simulink model "LV_grid"  (R2019b)
settings: Solver=VariableStepAuto  StartTime=0  StopTime=5.005  FixedStep=5e-4  RelTol=1e-3
model workspace (MAT data in the model file):
  P2_1 = 3450
libraries: powerlib x373, powerlib_meascontrol x37
(part 3 of 5)

== system LV_grid/L20 ==
  note: 2.5m
  note: 2.5m
  note: 2.5m
  Ground : powerlib/Elements/Ground  LConnTagsString=a
      settings: SourceProductName=Simscape Electrical
  Ground1 : powerlib/Elements/Ground  LConnTagsString=a
      settings: SourceProductName=Simscape Electrical
  L1 : Subsystem
  L2 : Subsystem
  L3 : Subsystem
  A : PMIOPort  Side=Left
  B : PMIOPort  Port=2  Side=Left
  C : PMIOPort  Port=3  Side=Left
  N : PMIOPort  Port=4  Side=Left
  a : PMIOPort  Port=5  Side=Right
  b : PMIOPort  Port=6  Side=Right
  c : PMIOPort  Port=7  Side=Right
  n : PMIOPort  Port=8  Side=Right
  connections:
  L1/LConn2 -- B/RConn1
  L1/LConn4 -- N/RConn1
  L1/LConn1 -- A/RConn1
  L1/RConn4 -- L2/LConn4 -- Ground/LConn1
  L1/LConn3 -- C/RConn1
  L3/RConn4 -- n/RConn1
  L2/RConn4 -- L3/LConn4 -- Ground1/LConn1
  L3/RConn1 -- a/RConn1
  L3/RConn2 -- b/RConn1
  L3/RConn3 -- c/RConn1
  L3/LConn1 -- L2/RConn1
  L3/LConn2 -- L2/RConn2
  L3/LConn3 -- L2/RConn3
  L2/LConn1 -- L1/RConn1
  L2/LConn2 -- L1/RConn2
  L2/LConn3 -- L1/RConn3

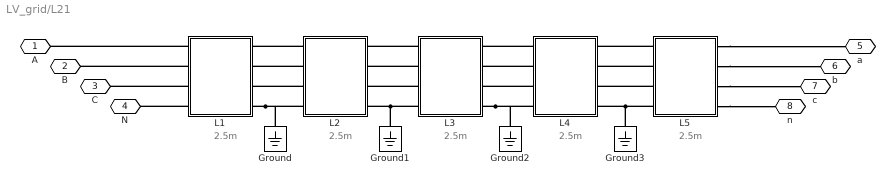
== system LV_grid/L21 ==
  note: 2.5m
  note: 2.5m
  note: 2.5m
  note: 2.5m
  note: 2.5m
  Ground{,1..3} (4 alike) : powerlib/Elements/Ground  LConnTagsString=a
      settings: SourceProductName=Simscape Electrical
  L1 : Subsystem
  L2 : Subsystem
  L3 : Subsystem
  L4 : Subsystem
  L5 : Subsystem
  A : PMIOPort  Side=Left
  B : PMIOPort  Port=2  Side=Left
  C : PMIOPort  Port=3  Side=Left
  N : PMIOPort  Port=4  Side=Left
  a : PMIOPort  Port=5  Side=Right
  b : PMIOPort  Port=6  Side=Right
  c : PMIOPort  Port=7  Side=Right
  n : PMIOPort  Port=8  Side=Right
  connections:
  L1/LConn1 -- A/RConn1
  L1/LConn4 -- N/RConn1
  L1/LConn2 -- B/RConn1
  L1/LConn3 -- C/RConn1
  L5/LConn4 -- L4/RConn4 -- Ground3/LConn1
  L3/RConn4 -- L4/LConn4 -- Ground2/LConn1
  L5/RConn4 -- n/RConn1
  L3/LConn4 -- L2/RConn4 -- Ground1/LConn1
  L1/RConn4 -- L2/LConn4 -- Ground/LConn1
  L5/RConn1 -- a/RConn1
  L5/RConn2 -- b/RConn1
  L5/RConn3 -- c/RConn1
  L2/LConn1 -- L1/RConn1
  L2/LConn2 -- L1/RConn2
  L2/LConn3 -- L1/RConn3
  L4/LConn1 -- L3/RConn1
  L4/LConn2 -- L3/RConn2
  L4/LConn3 -- L3/RConn3
  L5/LConn1 -- L4/RConn1
  L5/LConn2 -- L4/RConn2
  L5/LConn3 -- L4/RConn3
  L3/LConn1 -- L2/RConn1
  L3/LConn2 -- L2/RConn2
  L3/LConn3 -- L2/RConn3

== system LV_grid/L22 ==
  note: 2.5m
  note: 2.5m
  Ground : powerlib/Elements/Ground  LConnTagsString=a
      settings: SourceProductName=Simscape Electrical
  L1 : Subsystem
  L2 : Subsystem
  A : PMIOPort  Side=Left
  B : PMIOPort  Port=2  Side=Left
  C : PMIOPort  Port=3  Side=Left
  N : PMIOPort  Port=4  Side=Left
  a : PMIOPort  Port=5  Side=Right
  b : PMIOPort  Port=6  Side=Right
  c : PMIOPort  Port=7  Side=Right
  n : PMIOPort  Port=8  Side=Right
  connections:
  L2/RConn4 -- n/RConn1
  L1/RConn4 -- L2/LConn4 -- Ground/LConn1
  L1/LConn4 -- N/RConn1
  L1/LConn3 -- C/RConn1
  L1/LConn2 -- B/RConn1
  L1/LConn1 -- A/RConn1
  L2/LConn1 -- L1/RConn1
  L2/LConn2 -- L1/RConn2
  L2/LConn3 -- L1/RConn3
  L2/RConn1 -- a/RConn1
  L2/RConn2 -- b/RConn1
  L2/RConn3 -- c/RConn1

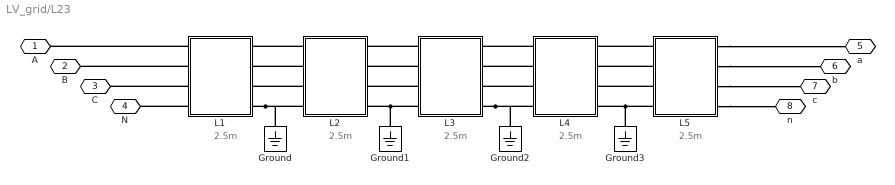
== system LV_grid/L23 ==
  note: 2.5m
  note: 2.5m
  note: 2.5m
  note: 2.5m
  note: 2.5m
  Ground{,1..3} (4 alike) : powerlib/Elements/Ground  LConnTagsString=a
      settings: SourceProductName=Simscape Electrical
  L1 : Subsystem
  L2 : Subsystem
  L3 : Subsystem
  L4 : Subsystem
  L5 : Subsystem
  A : PMIOPort  Side=Left
  B : PMIOPort  Port=2  Side=Left
  C : PMIOPort  Port=3  Side=Left
  N : PMIOPort  Port=4  Side=Left
  a : PMIOPort  Port=5  Side=Right
  b : PMIOPort  Port=6  Side=Right
  c : PMIOPort  Port=7  Side=Right
  n : PMIOPort  Port=8  Side=Right
  connections:
  L1/LConn1 -- A/RConn1
  L1/LConn4 -- N/RConn1
  L1/LConn2 -- B/RConn1
  L1/LConn3 -- C/RConn1
  L5/LConn4 -- L4/RConn4 -- Ground3/LConn1
  L3/RConn4 -- L4/LConn4 -- Ground2/LConn1
  L5/RConn4 -- n/RConn1
  L3/LConn4 -- L2/RConn4 -- Ground1/LConn1
  L1/RConn4 -- L2/LConn4 -- Ground/LConn1
  L4/LConn1 -- L3/RConn1
  L4/LConn2 -- L3/RConn2
  L4/LConn3 -- L3/RConn3
  L2/LConn1 -- L1/RConn1
  L2/LConn2 -- L1/RConn2
  L2/LConn3 -- L1/RConn3
  L5/RConn1 -- a/RConn1
  L5/RConn2 -- b/RConn1
  L5/RConn3 -- c/RConn1
  L5/LConn1 -- L4/RConn1
  L5/LConn2 -- L4/RConn2
  L5/LConn3 -- L4/RConn3
  L3/LConn1 -- L2/RConn1
  L3/LConn2 -- L2/RConn2
  L3/LConn3 -- L2/RConn3

== system LV_grid/L24 ==
  note: 2.5m
  note: 2.5m
  note: 2.5m
  note: 2.5m
  Ground : powerlib/Elements/Ground  LConnTagsString=a
      settings: SourceProductName=Simscape Electrical
  Ground1 : powerlib/Elements/Ground  LConnTagsString=a
      settings: SourceProductName=Simscape Electrical
  Ground2 : powerlib/Elements/Ground  LConnTagsString=a
      settings: SourceProductName=Simscape Electrical
  L1 : Subsystem
  L2 : Subsystem
  L3 : Subsystem
  L4 : Subsystem
  A : PMIOPort  Side=Left
  B : PMIOPort  Port=2  Side=Left
  C : PMIOPort  Port=3  Side=Left
  N : PMIOPort  Port=4  Side=Left
  a : PMIOPort  Port=5  Side=Right
  b : PMIOPort  Port=6  Side=Right
  c : PMIOPort  Port=7  Side=Right
  n : PMIOPort  Port=8  Side=Right
  connections:
  L1/LConn3 -- C/RConn1
  L2/RConn4 -- L3/LConn4 -- Ground1/LConn1
  L1/LConn4 -- N/RConn1
  L1/LConn2 -- B/RConn1
  L1/LConn1 -- A/RConn1
  L1/RConn4 -- L2/LConn4 -- Ground/LConn1
  L3/RConn4 -- L4/LConn4 -- Ground2/LConn1
  L4/RConn4 -- n/RConn1
  L4/RConn1 -- a/RConn1
  L4/RConn2 -- b/RConn1
  L4/RConn3 -- c/RConn1
  L3/LConn1 -- L2/RConn1
  L3/LConn2 -- L2/RConn2
  L3/LConn3 -- L2/RConn3
  L2/LConn1 -- L1/RConn1
  L2/LConn2 -- L1/RConn2
  L2/LConn3 -- L1/RConn3
  L4/LConn1 -- L3/RConn1
  L4/LConn2 -- L3/RConn2
  L4/LConn3 -- L3/RConn3

== system LV_grid/L25 ==
  note: 2.5m
  note: 2.5m
  note: 2.5m
  note: 2.5m
  Ground : powerlib/Elements/Ground  LConnTagsString=a
      settings: SourceProductName=Simscape Electrical
  Ground1 : powerlib/Elements/Ground  LConnTagsString=a
      settings: SourceProductName=Simscape Electrical
  Ground2 : powerlib/Elements/Ground  LConnTagsString=a
      settings: SourceProductName=Simscape Electrical
  L1 : Subsystem
  L2 : Subsystem
  L3 : Subsystem
  L4 : Subsystem
  A : PMIOPort  Side=Left
  B : PMIOPort  Port=2  Side=Left
  C : PMIOPort  Port=3  Side=Left
  N : PMIOPort  Port=4  Side=Left
  a : PMIOPort  Port=5  Side=Right
  b : PMIOPort  Port=6  Side=Right
  c : PMIOPort  Port=7  Side=Right
  n : PMIOPort  Port=8  Side=Right
  connections:
  L1/LConn3 -- C/RConn1
  L3/LConn4 -- Ground1/LConn1 -- L2/RConn4
  L1/LConn4 -- N/RConn1
  L1/LConn2 -- B/RConn1
  L1/LConn1 -- A/RConn1
  L2/LConn4 -- Ground/LConn1 -- L1/RConn4
  L4/LConn4 -- Ground2/LConn1 -- L3/RConn4
  L4/RConn4 -- n/RConn1
  L3/LConn1 -- L2/RConn1
  L3/LConn2 -- L2/RConn2
  L3/LConn3 -- L2/RConn3
  L4/LConn1 -- L3/RConn1
  L4/LConn2 -- L3/RConn2
  L4/LConn3 -- L3/RConn3
  L4/RConn1 -- a/RConn1
  L4/RConn2 -- b/RConn1
  L4/RConn3 -- c/RConn1
  L2/LConn1 -- L1/RConn1
  L2/LConn2 -- L1/RConn2
  L2/LConn3 -- L1/RConn3

== system LV_grid/L26 ==
  note: 2.5m
  note: 2.5m
  Ground : powerlib/Elements/Ground  LConnTagsString=a
      settings: SourceProductName=Simscape Electrical
  L1 : Subsystem
  L2 : Subsystem
  A : PMIOPort  Side=Left
  B : PMIOPort  Port=2  Side=Left
  C : PMIOPort  Port=3  Side=Left
  N : PMIOPort  Port=4  Side=Left
  a : PMIOPort  Port=5  Side=Right
  b : PMIOPort  Port=6  Side=Right
  c : PMIOPort  Port=7  Side=Right
  n : PMIOPort  Port=8  Side=Right
  connections:
  L2/RConn4 -- n/RConn1
  L1/RConn4 -- L2/LConn4 -- Ground/LConn1
  L1/LConn4 -- N/RConn1
  L1/LConn3 -- C/RConn1
  L1/LConn2 -- B/RConn1
  L1/LConn1 -- A/RConn1
  L2/RConn1 -- a/RConn1
  L2/RConn2 -- b/RConn1
  L2/RConn3 -- c/RConn1
  L2/LConn1 -- L1/RConn1
  L2/LConn2 -- L1/RConn2
  L2/LConn3 -- L1/RConn3

== system LV_grid/L27 ==
  note: 2.5m
  note: 2.5m
  Ground : powerlib/Elements/Ground  LConnTagsString=a
      settings: SourceProductName=Simscape Electrical
  L1 : Subsystem
  L2 : Subsystem
  A : PMIOPort  Side=Left
  B : PMIOPort  Port=2  Side=Left
  C : PMIOPort  Port=3  Side=Left
  N : PMIOPort  Port=4  Side=Left
  a : PMIOPort  Port=5  Side=Right
  b : PMIOPort  Port=6  Side=Right
  c : PMIOPort  Port=7  Side=Right
  n : PMIOPort  Port=8  Side=Right
  connections:
  L2/RConn4 -- n/RConn1
  L1/RConn4 -- L2/LConn4 -- Ground/LConn1
  L1/LConn4 -- N/RConn1
  L1/LConn3 -- C/RConn1
  L1/LConn2 -- B/RConn1
  L1/LConn1 -- A/RConn1
  L2/RConn1 -- a/RConn1
  L2/RConn2 -- b/RConn1
  L2/RConn3 -- c/RConn1
  L2/LConn1 -- L1/RConn1
  L2/LConn2 -- L1/RConn2
  L2/LConn3 -- L1/RConn3

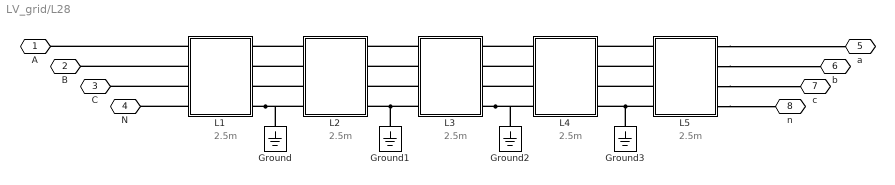
== system LV_grid/L28 ==
  note: 2.5m
  note: 2.5m
  note: 2.5m
  note: 2.5m
  note: 2.5m
  Ground{,1..3} (4 alike) : powerlib/Elements/Ground  LConnTagsString=a
      settings: SourceProductName=Simscape Electrical
  L1 : Subsystem
  L2 : Subsystem
  L3 : Subsystem
  L4 : Subsystem
  L5 : Subsystem
  A : PMIOPort  Side=Left
  B : PMIOPort  Port=2  Side=Left
  C : PMIOPort  Port=3  Side=Left
  N : PMIOPort  Port=4  Side=Left
  a : PMIOPort  Port=5  Side=Right
  b : PMIOPort  Port=6  Side=Right
  c : PMIOPort  Port=7  Side=Right
  n : PMIOPort  Port=8  Side=Right
  connections:
  L1/LConn1 -- A/RConn1
  L1/LConn4 -- N/RConn1
  L1/LConn2 -- B/RConn1
  L1/LConn3 -- C/RConn1
  L5/LConn4 -- L4/RConn4 -- Ground3/LConn1
  L3/RConn4 -- L4/LConn4 -- Ground2/LConn1
  L5/RConn4 -- n/RConn1
  L3/LConn4 -- L2/RConn4 -- Ground1/LConn1
  L1/RConn4 -- L2/LConn4 -- Ground/LConn1
  L3/LConn1 -- L2/RConn1
  L3/LConn2 -- L2/RConn2
  L3/LConn3 -- L2/RConn3
  L5/RConn1 -- a/RConn1
  L5/RConn2 -- b/RConn1
  L5/RConn3 -- c/RConn1
  L5/LConn1 -- L4/RConn1
  L5/LConn2 -- L4/RConn2
  L5/LConn3 -- L4/RConn3
  L4/LConn1 -- L3/RConn1
  L4/LConn2 -- L3/RConn2
  L4/LConn3 -- L3/RConn3
  L2/LConn1 -- L1/RConn1
  L2/LConn2 -- L1/RConn2
  L2/LConn3 -- L1/RConn3

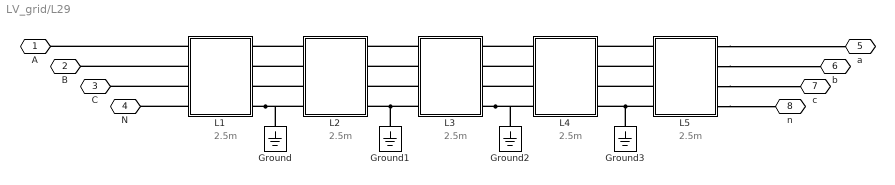
== system LV_grid/L29 ==
  note: 2.5m
  note: 2.5m
  note: 2.5m
  note: 2.5m
  note: 2.5m
  Ground{,1..3} (4 alike) : powerlib/Elements/Ground  LConnTagsString=a
      settings: SourceProductName=Simscape Electrical
  L1 : Subsystem
  L2 : Subsystem
  L3 : Subsystem
  L4 : Subsystem
  L5 : Subsystem
  A : PMIOPort  Side=Left
  B : PMIOPort  Port=2  Side=Left
  C : PMIOPort  Port=3  Side=Left
  N : PMIOPort  Port=4  Side=Left
  a : PMIOPort  Port=5  Side=Right
  b : PMIOPort  Port=6  Side=Right
  c : PMIOPort  Port=7  Side=Right
  n : PMIOPort  Port=8  Side=Right
  connections:
  L1/LConn1 -- A/RConn1
  L1/LConn4 -- N/RConn1
  L1/LConn2 -- B/RConn1
  L1/LConn3 -- C/RConn1
  L5/LConn4 -- L4/RConn4 -- Ground3/LConn1
  L3/RConn4 -- L4/LConn4 -- Ground2/LConn1
  L5/RConn4 -- n/RConn1
  L3/LConn4 -- L2/RConn4 -- Ground1/LConn1
  L1/RConn4 -- L2/LConn4 -- Ground/LConn1
  L4/LConn1 -- L3/RConn1
  L4/LConn2 -- L3/RConn2
  L4/LConn3 -- L3/RConn3
  L5/LConn1 -- L4/RConn1
  L5/LConn2 -- L4/RConn2
  L5/LConn3 -- L4/RConn3
  L2/LConn1 -- L1/RConn1
  L2/LConn2 -- L1/RConn2
  L2/LConn3 -- L1/RConn3
  L5/RConn1 -- a/RConn1
  L5/RConn2 -- b/RConn1
  L5/RConn3 -- c/RConn1
  L3/LConn1 -- L2/RConn1
  L3/LConn2 -- L2/RConn2
  L3/LConn3 -- L2/RConn3

== system LV_grid/L3 ==
  note: 2.5m
  L1 : Subsystem
  A : PMIOPort  Side=Left
  B : PMIOPort  Port=2  Side=Left
  C : PMIOPort  Port=3  Side=Left
  N : PMIOPort  Port=4  Side=Left
  a : PMIOPort  Port=5  Side=Right
  b : PMIOPort  Port=6  Side=Right
  c : PMIOPort  Port=7  Side=Right
  n : PMIOPort  Port=8  Side=Right
  connections:
  B/RConn1 -- L1/LConn2
  n/RConn1 -- L1/RConn4
  C/RConn1 -- L1/LConn3
  N/RConn1 -- L1/LConn4
  A/RConn1 -- L1/LConn1
  L1/RConn1 -- a/RConn1
  L1/RConn2 -- b/RConn1
  L1/RConn3 -- c/RConn1

== system LV_grid/L30 ==
  note: 2.5m
  note: 2.5m
  Ground : powerlib/Elements/Ground  LConnTagsString=a
      settings: SourceProductName=Simscape Electrical
  L1 : Subsystem
  L2 : Subsystem
  A : PMIOPort  Side=Left
  B : PMIOPort  Port=2  Side=Left
  C : PMIOPort  Port=3  Side=Left
  N : PMIOPort  Port=4  Side=Left
  a : PMIOPort  Port=5  Side=Right
  b : PMIOPort  Port=6  Side=Right
  c : PMIOPort  Port=7  Side=Right
  n : PMIOPort  Port=8  Side=Right
  connections:
  L2/RConn4 -- n/RConn1
  L1/RConn4 -- L2/LConn4 -- Ground/LConn1
  L1/LConn4 -- N/RConn1
  L1/LConn3 -- C/RConn1
  L1/LConn2 -- B/RConn1
  L1/LConn1 -- A/RConn1
  L2/LConn1 -- L1/RConn1
  L2/LConn2 -- L1/RConn2
  L2/LConn3 -- L1/RConn3
  L2/RConn1 -- a/RConn1
  L2/RConn2 -- b/RConn1
  L2/RConn3 -- c/RConn1

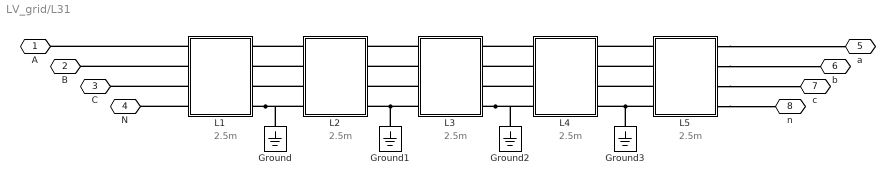
== system LV_grid/L31 ==
  note: 2.5m
  note: 2.5m
  note: 2.5m
  note: 2.5m
  note: 2.5m
  Ground{,1..3} (4 alike) : powerlib/Elements/Ground  LConnTagsString=a
      settings: SourceProductName=Simscape Electrical
  L1 : Subsystem
  L2 : Subsystem
  L3 : Subsystem
  L4 : Subsystem
  L5 : Subsystem
  A : PMIOPort  Side=Left
  B : PMIOPort  Port=2  Side=Left
  C : PMIOPort  Port=3  Side=Left
  N : PMIOPort  Port=4  Side=Left
  a : PMIOPort  Port=5  Side=Right
  b : PMIOPort  Port=6  Side=Right
  c : PMIOPort  Port=7  Side=Right
  n : PMIOPort  Port=8  Side=Right
  connections:
  L1/LConn1 -- A/RConn1
  L1/LConn4 -- N/RConn1
  L1/LConn2 -- B/RConn1
  L1/LConn3 -- C/RConn1
  L5/LConn4 -- L4/RConn4 -- Ground3/LConn1
  L3/RConn4 -- L4/LConn4 -- Ground2/LConn1
  L5/RConn4 -- n/RConn1
  L3/LConn4 -- L2/RConn4 -- Ground1/LConn1
  L1/RConn4 -- L2/LConn4 -- Ground/LConn1
  L5/RConn1 -- a/RConn1
  L5/RConn2 -- b/RConn1
  L5/RConn3 -- c/RConn1
  L3/LConn1 -- L2/RConn1
  L3/LConn2 -- L2/RConn2
  L3/LConn3 -- L2/RConn3
  L2/LConn1 -- L1/RConn1
  L2/LConn2 -- L1/RConn2
  L2/LConn3 -- L1/RConn3
  L5/LConn1 -- L4/RConn1
  L5/LConn2 -- L4/RConn2
  L5/LConn3 -- L4/RConn3
  L4/LConn1 -- L3/RConn1
  L4/LConn2 -- L3/RConn2
  L4/LConn3 -- L3/RConn3

== system LV_grid/L32 ==
  note: 2.5m
  note: 2.5m
  note: 2.5m
  note: 2.5m
  Ground : powerlib/Elements/Ground  LConnTagsString=a
      settings: SourceProductName=Simscape Electrical
  Ground1 : powerlib/Elements/Ground  LConnTagsString=a
      settings: SourceProductName=Simscape Electrical
  Ground2 : powerlib/Elements/Ground  LConnTagsString=a
      settings: SourceProductName=Simscape Electrical
  L1 : Subsystem
  L2 : Subsystem
  L3 : Subsystem
  L4 : Subsystem
  A : PMIOPort  Side=Left
  B : PMIOPort  Port=2  Side=Left
  C : PMIOPort  Port=3  Side=Left
  N : PMIOPort  Port=4  Side=Left
  a : PMIOPort  Port=5  Side=Right
  b : PMIOPort  Port=6  Side=Right
  c : PMIOPort  Port=7  Side=Right
  n : PMIOPort  Port=8  Side=Right
  connections:
  L1/LConn3 -- C/RConn1
  L2/RConn4 -- L3/LConn4 -- Ground1/LConn1
  L1/LConn4 -- N/RConn1
  L1/LConn2 -- B/RConn1
  L1/LConn1 -- A/RConn1
  L1/RConn4 -- L2/LConn4 -- Ground/LConn1
  L3/RConn4 -- L4/LConn4 -- Ground2/LConn1
  L4/RConn4 -- n/RConn1
  L4/RConn1 -- a/RConn1
  L4/RConn2 -- b/RConn1
  L4/RConn3 -- c/RConn1
  L2/LConn1 -- L1/RConn1
  L2/LConn2 -- L1/RConn2
  L2/LConn3 -- L1/RConn3
  L4/LConn1 -- L3/RConn1
  L4/LConn2 -- L3/RConn2
  L4/LConn3 -- L3/RConn3
  L3/LConn1 -- L2/RConn1
  L3/LConn2 -- L2/RConn2
  L3/LConn3 -- L2/RConn3

== system LV_grid/L4 ==
  note: 2.5m
  note: 2.5m
  Ground : powerlib/Elements/Ground  LConnTagsString=a
      settings: SourceProductName=Simscape Electrical
  L1 : Subsystem
  L2 : Subsystem
  A : PMIOPort  Side=Left
  B : PMIOPort  Port=2  Side=Left
  C : PMIOPort  Port=3  Side=Left
  N : PMIOPort  Port=4  Side=Left
  a : PMIOPort  Port=5  Side=Right
  b : PMIOPort  Port=6  Side=Right
  c : PMIOPort  Port=7  Side=Right
  n : PMIOPort  Port=8  Side=Right
  connections:
  L2/RConn4 -- n/RConn1
  L2/LConn4 -- Ground/LConn1 -- L1/RConn4
  L1/LConn4 -- N/RConn1
  L1/LConn3 -- C/RConn1
  L1/LConn2 -- B/RConn1
  L1/LConn1 -- A/RConn1
  L2/LConn1 -- L1/RConn1
  L2/LConn2 -- L1/RConn2
  L2/LConn3 -- L1/RConn3
  L2/RConn1 -- a/RConn1
  L2/RConn2 -- b/RConn1
  L2/RConn3 -- c/RConn1

== system LV_grid/L5 ==
  note: 2.5m
  note: 2.5m
  Ground : powerlib/Elements/Ground  LConnTagsString=a
      settings: SourceProductName=Simscape Electrical
  L1 : Subsystem
  L2 : Subsystem
  A : PMIOPort  Side=Left
  B : PMIOPort  Port=2  Side=Left
  C : PMIOPort  Port=3  Side=Left
  N : PMIOPort  Port=4  Side=Left
  a : PMIOPort  Port=5  Side=Right
  b : PMIOPort  Port=6  Side=Right
  c : PMIOPort  Port=7  Side=Right
  n : PMIOPort  Port=8  Side=Right
  connections:
  L2/RConn4 -- n/RConn1
  L1/RConn4 -- L2/LConn4 -- Ground/LConn1
  L1/LConn4 -- N/RConn1
  L1/LConn3 -- C/RConn1
  L1/LConn2 -- B/RConn1
  L1/LConn1 -- A/RConn1
  L2/LConn1 -- L1/RConn1
  L2/LConn2 -- L1/RConn2
  L2/LConn3 -- L1/RConn3
  L2/RConn1 -- a/RConn1
  L2/RConn2 -- b/RConn1
  L2/RConn3 -- c/RConn1

== system LV_grid/L6 ==
  note: 2.5m
  L1 : Subsystem
  A : PMIOPort  Side=Left
  B : PMIOPort  Port=2  Side=Left
  C : PMIOPort  Port=3  Side=Left
  N : PMIOPort  Port=4  Side=Left
  a : PMIOPort  Port=5  Side=Right
  b : PMIOPort  Port=6  Side=Right
  c : PMIOPort  Port=7  Side=Right
  n : PMIOPort  Port=8  Side=Right
  connections:
  B/RConn1 -- L1/LConn2
  n/RConn1 -- L1/RConn4
  C/RConn1 -- L1/LConn3
  N/RConn1 -- L1/LConn4
  A/RConn1 -- L1/LConn1
  L1/RConn1 -- a/RConn1
  L1/RConn2 -- b/RConn1
  L1/RConn3 -- c/RConn1

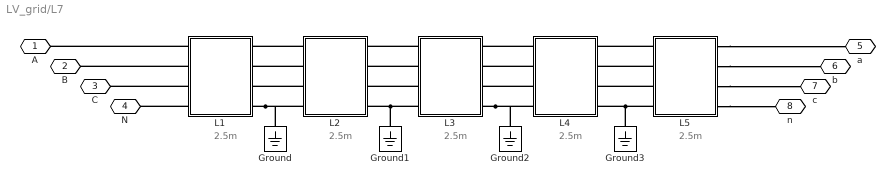
== system LV_grid/L7 ==
  note: 2.5m
  note: 2.5m
  note: 2.5m
  note: 2.5m
  note: 2.5m
  Ground{,1..3} (4 alike) : powerlib/Elements/Ground  LConnTagsString=a
      settings: SourceProductName=Simscape Electrical
  L1 : Subsystem
  L2 : Subsystem
  L3 : Subsystem
  L4 : Subsystem
  L5 : Subsystem
  A : PMIOPort  Side=Left
  B : PMIOPort  Port=2  Side=Left
  C : PMIOPort  Port=3  Side=Left
  N : PMIOPort  Port=4  Side=Left
  a : PMIOPort  Port=5  Side=Right
  b : PMIOPort  Port=6  Side=Right
  c : PMIOPort  Port=7  Side=Right
  n : PMIOPort  Port=8  Side=Right
  connections:
  L1/LConn1 -- A/RConn1
  L1/LConn4 -- N/RConn1
  L1/LConn2 -- B/RConn1
  L1/LConn3 -- C/RConn1
  L5/LConn4 -- L4/RConn4 -- Ground3/LConn1
  L3/RConn4 -- L4/LConn4 -- Ground2/LConn1
  L5/RConn4 -- n/RConn1
  L3/LConn4 -- L2/RConn4 -- Ground1/LConn1
  L1/RConn4 -- L2/LConn4 -- Ground/LConn1
  L3/LConn1 -- L2/RConn1
  L3/LConn2 -- L2/RConn2
  L3/LConn3 -- L2/RConn3
  L5/LConn1 -- L4/RConn1
  L5/LConn2 -- L4/RConn2
  L5/LConn3 -- L4/RConn3
  L5/RConn1 -- a/RConn1
  L5/RConn2 -- b/RConn1
  L5/RConn3 -- c/RConn1
  L4/LConn1 -- L3/RConn1
  L4/LConn2 -- L3/RConn2
  L4/LConn3 -- L3/RConn3
  L2/LConn1 -- L1/RConn1
  L2/LConn2 -- L1/RConn2
  L2/LConn3 -- L1/RConn3

== system LV_grid/L8 ==
  note: 2.5m
  note: 2.5m
  note: 2.5m
  Ground : powerlib/Elements/Ground  LConnTagsString=a
      settings: SourceProductName=Simscape Electrical
  Ground1 : powerlib/Elements/Ground  LConnTagsString=a
      settings: SourceProductName=Simscape Electrical
  L1 : Subsystem
  L2 : Subsystem
  L3 : Subsystem
  A : PMIOPort  Side=Left
  B : PMIOPort  Port=2  Side=Left
  C : PMIOPort  Port=3  Side=Left
  N : PMIOPort  Port=4  Side=Left
  a : PMIOPort  Port=5  Side=Right
  b : PMIOPort  Port=6  Side=Right
  c : PMIOPort  Port=7  Side=Right
  n : PMIOPort  Port=8  Side=Right
  connections:
  L1/LConn2 -- B/RConn1
  L1/LConn4 -- N/RConn1
  L1/LConn1 -- A/RConn1
  L2/LConn4 -- Ground/LConn1 -- L1/RConn4
  L1/LConn3 -- C/RConn1
  L3/RConn4 -- n/RConn1
  L3/LConn4 -- Ground1/LConn1 -- L2/RConn4
  L3/RConn1 -- a/RConn1
  L3/RConn2 -- b/RConn1
  L3/RConn3 -- c/RConn1
  L3/LConn1 -- L2/RConn1
  L3/LConn2 -- L2/RConn2
  L3/LConn3 -- L2/RConn3
  L2/LConn1 -- L1/RConn1
  L2/LConn2 -- L1/RConn2
  L2/LConn3 -- L1/RConn3

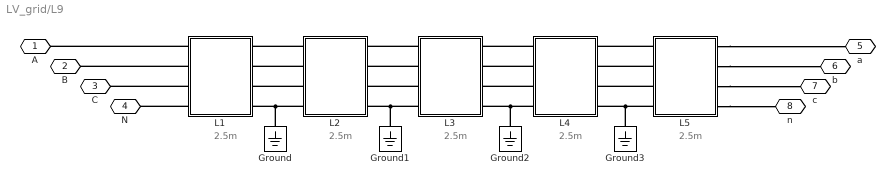
== system LV_grid/L9 ==
  note: 2.5m
  note: 2.5m
  note: 2.5m
  note: 2.5m
  note: 2.5m
  Ground{,1..3} (4 alike) : powerlib/Elements/Ground  LConnTagsString=a
      settings: SourceProductName=Simscape Electrical
  L1 : Subsystem
  L2 : Subsystem
  L3 : Subsystem
  L4 : Subsystem
  L5 : Subsystem
  A : PMIOPort  Side=Left
  B : PMIOPort  Port=2  Side=Left
  C : PMIOPort  Port=3  Side=Left
  N : PMIOPort  Port=4  Side=Left
  a : PMIOPort  Port=5  Side=Right
  b : PMIOPort  Port=6  Side=Right
  c : PMIOPort  Port=7  Side=Right
  n : PMIOPort  Port=8  Side=Right
  connections:
  L1/LConn1 -- A/RConn1
  L1/LConn4 -- N/RConn1
  L1/LConn2 -- B/RConn1
  L1/LConn3 -- C/RConn1
  L5/LConn4 -- Ground3/LConn1 -- L4/RConn4
  L4/LConn4 -- Ground2/LConn1 -- L3/RConn4
  L5/RConn4 -- n/RConn1
  L3/LConn4 -- Ground1/LConn1 -- L2/RConn4
  L2/LConn4 -- Ground/LConn1 -- L1/RConn4
  L5/LConn1 -- L4/RConn1
  L5/LConn2 -- L4/RConn2
  L5/LConn3 -- L4/RConn3
  L5/RConn1 -- a/RConn1
  L5/RConn2 -- b/RConn1
  L5/RConn3 -- c/RConn1
  L4/LConn1 -- L3/RConn1
  L4/LConn2 -- L3/RConn2
  L4/LConn3 -- L3/RConn3
  L2/LConn1 -- L1/RConn1
  L2/LConn2 -- L1/RConn2
  L2/LConn3 -- L1/RConn3
  L3/LConn1 -- L2/RConn1
  L3/LConn2 -- L2/RConn2
  L3/LConn3 -- L2/RConn3

== system LV_grid/L1/L1 ==
  Pi Section Line : powerlib/Elements/Pi Section Line  LConnTagsString=__new0  RConnTagsString=__new0  Frequency=50  Resistance=0.274  Inductance=0.073  Capacitance=12.74e-9  Length=0.0025  PiSections=1  Measurements=None
      settings: AttributesFormatString=\n  SourceProductName=Simscape Electrical  SourceProductBaseCode=PS
  Three-Phase PI Section Line : powerlib/Elements/Three-Phase PI Section Line  LConnTagsString=a|b|c  RConnTagsString=A|B|C  Frequency=50  Resistances=[ 0.274 0.959]  Inductances=[ 0.073 0.079]  Capacitances=[12.74e-9 7.751e-9]  Length=0.0025
      settings: SourceProductName=Simscape Electrical
  A : PMIOPort  Side=Left
  B : PMIOPort  Port=2  Side=Left
  C : PMIOPort  Port=3  Side=Left
  N : PMIOPort  Port=4  Side=Left
  a : PMIOPort  Port=5  Side=Right
  b : PMIOPort  Port=6  Side=Right
  c : PMIOPort  Port=7  Side=Right
  n : PMIOPort  Port=8  Side=Right
  connections:
  Pi Section Line/LConn1 -- N/RConn1
  Pi Section Line/RConn1 -- n/RConn1
  C/RConn1 -- Three-Phase PI Section Line/LConn3
  B/RConn1 -- Three-Phase PI Section Line/LConn2
  A/RConn1 -- Three-Phase PI Section Line/LConn1
  Three-Phase PI Section Line/RConn3 -- c/RConn1
  Three-Phase PI Section Line/RConn2 -- b/RConn1
  Three-Phase PI Section Line/RConn1 -- a/RConn1

== system LV_grid/L10/L1 ==
  Pi Section Line : powerlib/Elements/Pi Section Line  LConnTagsString=__new0  RConnTagsString=__new0  Frequency=50  Resistance=0.274  Inductance=0.073  Capacitance=12.74e-9  Length=0.0025  PiSections=1  Measurements=None
      settings: AttributesFormatString=\n  SourceProductName=Simscape Electrical  SourceProductBaseCode=PS
  Three-Phase PI Section Line : powerlib/Elements/Three-Phase PI Section Line  LConnTagsString=a|b|c  RConnTagsString=A|B|C  Frequency=50  Resistances=[ 0.274 0.959]  Inductances=[ 0.073 0.079]  Capacitances=[12.74e-9 7.751e-9]  Length=0.0025
      settings: SourceProductName=Simscape Electrical
  A : PMIOPort  Side=Left
  B : PMIOPort  Port=2  Side=Left
  C : PMIOPort  Port=3  Side=Left
  N : PMIOPort  Port=4  Side=Left
  a : PMIOPort  Port=5  Side=Right
  b : PMIOPort  Port=6  Side=Right
  c : PMIOPort  Port=7  Side=Right
  n : PMIOPort  Port=8  Side=Right
  connections:
  Pi Section Line/LConn1 -- N/RConn1
  Pi Section Line/RConn1 -- n/RConn1
  C/RConn1 -- Three-Phase PI Section Line/LConn3
  B/RConn1 -- Three-Phase PI Section Line/LConn2
  A/RConn1 -- Three-Phase PI Section Line/LConn1
  Three-Phase PI Section Line/RConn3 -- c/RConn1
  Three-Phase PI Section Line/RConn2 -- b/RConn1
  Three-Phase PI Section Line/RConn1 -- a/RConn1

== system LV_grid/L10/L2 ==
  Pi Section Line : powerlib/Elements/Pi Section Line  LConnTagsString=__new0  RConnTagsString=__new0  Frequency=50  Resistance=0.274  Inductance=0.073  Capacitance=12.74e-9  Length=0.0025  PiSections=1  Measurements=None
      settings: AttributesFormatString=\n  SourceProductName=Simscape Electrical  SourceProductBaseCode=PS
  Three-Phase PI Section Line : powerlib/Elements/Three-Phase PI Section Line  LConnTagsString=a|b|c  RConnTagsString=A|B|C  Frequency=50  Resistances=[ 0.274 0.959]  Inductances=[ 0.073 0.079]  Capacitances=[12.74e-9 7.751e-9]  Length=0.0025
      settings: SourceProductName=Simscape Electrical
  A : PMIOPort  Side=Left
  B : PMIOPort  Port=2  Side=Left
  C : PMIOPort  Port=3  Side=Left
  N : PMIOPort  Port=4  Side=Left
  a : PMIOPort  Port=5  Side=Right
  b : PMIOPort  Port=6  Side=Right
  c : PMIOPort  Port=7  Side=Right
  n : PMIOPort  Port=8  Side=Right
  connections:
  Pi Section Line/LConn1 -- N/RConn1
  Pi Section Line/RConn1 -- n/RConn1
  C/RConn1 -- Three-Phase PI Section Line/LConn3
  B/RConn1 -- Three-Phase PI Section Line/LConn2
  A/RConn1 -- Three-Phase PI Section Line/LConn1
  Three-Phase PI Section Line/RConn3 -- c/RConn1
  Three-Phase PI Section Line/RConn2 -- b/RConn1
  Three-Phase PI Section Line/RConn1 -- a/RConn1

== system LV_grid/L11/L1 ==
  Pi Section Line : powerlib/Elements/Pi Section Line  LConnTagsString=__new0  RConnTagsString=__new0  Frequency=50  Resistance=0.274  Inductance=0.073  Capacitance=12.74e-9  Length=0.0025  PiSections=1  Measurements=None
      settings: AttributesFormatString=\n  SourceProductName=Simscape Electrical  SourceProductBaseCode=PS
  Three-Phase PI Section Line : powerlib/Elements/Three-Phase PI Section Line  LConnTagsString=a|b|c  RConnTagsString=A|B|C  Frequency=50  Resistances=[ 0.274 0.959]  Inductances=[ 0.073 0.079]  Capacitances=[12.74e-9 7.751e-9]  Length=0.0025
      settings: SourceProductName=Simscape Electrical
  A : PMIOPort  Side=Left
  B : PMIOPort  Port=2  Side=Left
  C : PMIOPort  Port=3  Side=Left
  N : PMIOPort  Port=4  Side=Left
  a : PMIOPort  Port=5  Side=Right
  b : PMIOPort  Port=6  Side=Right
  c : PMIOPort  Port=7  Side=Right
  n : PMIOPort  Port=8  Side=Right
  connections:
  Pi Section Line/LConn1 -- N/RConn1
  Pi Section Line/RConn1 -- n/RConn1
  C/RConn1 -- Three-Phase PI Section Line/LConn3
  B/RConn1 -- Three-Phase PI Section Line/LConn2
  A/RConn1 -- Three-Phase PI Section Line/LConn1
  Three-Phase PI Section Line/RConn3 -- c/RConn1
  Three-Phase PI Section Line/RConn2 -- b/RConn1
  Three-Phase PI Section Line/RConn1 -- a/RConn1

== system LV_grid/L11/L2 ==
  Pi Section Line : powerlib/Elements/Pi Section Line  LConnTagsString=__new0  RConnTagsString=__new0  Frequency=50  Resistance=0.274  Inductance=0.073  Capacitance=12.74e-9  Length=0.0025  PiSections=1  Measurements=None
      settings: AttributesFormatString=\n  SourceProductName=Simscape Electrical  SourceProductBaseCode=PS
  Three-Phase PI Section Line : powerlib/Elements/Three-Phase PI Section Line  LConnTagsString=a|b|c  RConnTagsString=A|B|C  Frequency=50  Resistances=[ 0.274 0.959]  Inductances=[ 0.073 0.079]  Capacitances=[12.74e-9 7.751e-9]  Length=0.0025
      settings: SourceProductName=Simscape Electrical
  A : PMIOPort  Side=Left
  B : PMIOPort  Port=2  Side=Left
  C : PMIOPort  Port=3  Side=Left
  N : PMIOPort  Port=4  Side=Left
  a : PMIOPort  Port=5  Side=Right
  b : PMIOPort  Port=6  Side=Right
  c : PMIOPort  Port=7  Side=Right
  n : PMIOPort  Port=8  Side=Right
  connections:
  Pi Section Line/LConn1 -- N/RConn1
  Pi Section Line/RConn1 -- n/RConn1
  C/RConn1 -- Three-Phase PI Section Line/LConn3
  B/RConn1 -- Three-Phase PI Section Line/LConn2
  A/RConn1 -- Three-Phase PI Section Line/LConn1
  Three-Phase PI Section Line/RConn3 -- c/RConn1
  Three-Phase PI Section Line/RConn2 -- b/RConn1
  Three-Phase PI Section Line/RConn1 -- a/RConn1

== system LV_grid/L12/L1 ==
  Pi Section Line : powerlib/Elements/Pi Section Line  LConnTagsString=__new0  RConnTagsString=__new0  Frequency=50  Resistance=0.274  Inductance=0.073  Capacitance=12.74e-9  Length=0.0025  PiSections=1  Measurements=None
      settings: AttributesFormatString=\n  SourceProductName=Simscape Electrical  SourceProductBaseCode=PS
  Three-Phase PI Section Line : powerlib/Elements/Three-Phase PI Section Line  LConnTagsString=a|b|c  RConnTagsString=A|B|C  Frequency=50  Resistances=[ 0.274 0.959]  Inductances=[ 0.073 0.079]  Capacitances=[12.74e-9 7.751e-9]  Length=0.0025
      settings: SourceProductName=Simscape Electrical
  A : PMIOPort  Side=Left
  B : PMIOPort  Port=2  Side=Left
  C : PMIOPort  Port=3  Side=Left
  N : PMIOPort  Port=4  Side=Left
  a : PMIOPort  Port=5  Side=Right
  b : PMIOPort  Port=6  Side=Right
  c : PMIOPort  Port=7  Side=Right
  n : PMIOPort  Port=8  Side=Right
  connections:
  Pi Section Line/LConn1 -- N/RConn1
  Pi Section Line/RConn1 -- n/RConn1
  C/RConn1 -- Three-Phase PI Section Line/LConn3
  B/RConn1 -- Three-Phase PI Section Line/LConn2
  A/RConn1 -- Three-Phase PI Section Line/LConn1
  Three-Phase PI Section Line/RConn3 -- c/RConn1
  Three-Phase PI Section Line/RConn2 -- b/RConn1
  Three-Phase PI Section Line/RConn1 -- a/RConn1

== system LV_grid/L12/L2 ==
  Pi Section Line : powerlib/Elements/Pi Section Line  LConnTagsString=__new0  RConnTagsString=__new0  Frequency=50  Resistance=0.274  Inductance=0.073  Capacitance=12.74e-9  Length=0.0025  PiSections=1  Measurements=None
      settings: AttributesFormatString=\n  SourceProductName=Simscape Electrical  SourceProductBaseCode=PS
  Three-Phase PI Section Line : powerlib/Elements/Three-Phase PI Section Line  LConnTagsString=a|b|c  RConnTagsString=A|B|C  Frequency=50  Resistances=[ 0.274 0.959]  Inductances=[ 0.073 0.079]  Capacitances=[12.74e-9 7.751e-9]  Length=0.0025
      settings: SourceProductName=Simscape Electrical
  A : PMIOPort  Side=Left
  B : PMIOPort  Port=2  Side=Left
  C : PMIOPort  Port=3  Side=Left
  N : PMIOPort  Port=4  Side=Left
  a : PMIOPort  Port=5  Side=Right
  b : PMIOPort  Port=6  Side=Right
  c : PMIOPort  Port=7  Side=Right
  n : PMIOPort  Port=8  Side=Right
  connections:
  Pi Section Line/LConn1 -- N/RConn1
  Pi Section Line/RConn1 -- n/RConn1
  C/RConn1 -- Three-Phase PI Section Line/LConn3
  B/RConn1 -- Three-Phase PI Section Line/LConn2
  A/RConn1 -- Three-Phase PI Section Line/LConn1
  Three-Phase PI Section Line/RConn3 -- c/RConn1
  Three-Phase PI Section Line/RConn2 -- b/RConn1
  Three-Phase PI Section Line/RConn1 -- a/RConn1

== system LV_grid/L12/L3 ==
  Pi Section Line : powerlib/Elements/Pi Section Line  LConnTagsString=__new0  RConnTagsString=__new0  Frequency=50  Resistance=0.274  Inductance=0.073  Capacitance=12.74e-9  Length=0.0025  PiSections=1  Measurements=None
      settings: AttributesFormatString=\n  SourceProductName=Simscape Electrical  SourceProductBaseCode=PS
  Three-Phase PI Section Line : powerlib/Elements/Three-Phase PI Section Line  LConnTagsString=a|b|c  RConnTagsString=A|B|C  Frequency=50  Resistances=[ 0.274 0.959]  Inductances=[ 0.073 0.079]  Capacitances=[12.74e-9 7.751e-9]  Length=0.0025
      settings: SourceProductName=Simscape Electrical
  A : PMIOPort  Side=Left
  B : PMIOPort  Port=2  Side=Left
  C : PMIOPort  Port=3  Side=Left
  N : PMIOPort  Port=4  Side=Left
  a : PMIOPort  Port=5  Side=Right
  b : PMIOPort  Port=6  Side=Right
  c : PMIOPort  Port=7  Side=Right
  n : PMIOPort  Port=8  Side=Right
  connections:
  Pi Section Line/LConn1 -- N/RConn1
  Pi Section Line/RConn1 -- n/RConn1
  C/RConn1 -- Three-Phase PI Section Line/LConn3
  B/RConn1 -- Three-Phase PI Section Line/LConn2
  A/RConn1 -- Three-Phase PI Section Line/LConn1
  Three-Phase PI Section Line/RConn3 -- c/RConn1
  Three-Phase PI Section Line/RConn2 -- b/RConn1
  Three-Phase PI Section Line/RConn1 -- a/RConn1

== system LV_grid/L12/L4 ==
  Pi Section Line : powerlib/Elements/Pi Section Line  LConnTagsString=__new0  RConnTagsString=__new0  Frequency=50  Resistance=0.274  Inductance=0.073  Capacitance=12.74e-9  Length=0.0025  PiSections=1  Measurements=None
      settings: AttributesFormatString=\n  SourceProductName=Simscape Electrical  SourceProductBaseCode=PS
  Three-Phase PI Section Line : powerlib/Elements/Three-Phase PI Section Line  LConnTagsString=a|b|c  RConnTagsString=A|B|C  Frequency=50  Resistances=[ 0.274 0.959]  Inductances=[ 0.073 0.079]  Capacitances=[12.74e-9 7.751e-9]  Length=0.0025
      settings: SourceProductName=Simscape Electrical
  A : PMIOPort  Side=Left
  B : PMIOPort  Port=2  Side=Left
  C : PMIOPort  Port=3  Side=Left
  N : PMIOPort  Port=4  Side=Left
  a : PMIOPort  Port=5  Side=Right
  b : PMIOPort  Port=6  Side=Right
  c : PMIOPort  Port=7  Side=Right
  n : PMIOPort  Port=8  Side=Right
  connections:
  Pi Section Line/LConn1 -- N/RConn1
  Pi Section Line/RConn1 -- n/RConn1
  C/RConn1 -- Three-Phase PI Section Line/LConn3
  B/RConn1 -- Three-Phase PI Section Line/LConn2
  A/RConn1 -- Three-Phase PI Section Line/LConn1
  Three-Phase PI Section Line/RConn3 -- c/RConn1
  Three-Phase PI Section Line/RConn2 -- b/RConn1
  Three-Phase PI Section Line/RConn1 -- a/RConn1

== system LV_grid/L12/L5 ==
  Pi Section Line : powerlib/Elements/Pi Section Line  LConnTagsString=__new0  RConnTagsString=__new0  Frequency=50  Resistance=0.274  Inductance=0.073  Capacitance=12.74e-9  Length=0.0025  PiSections=1  Measurements=None
      settings: AttributesFormatString=\n  SourceProductName=Simscape Electrical  SourceProductBaseCode=PS
  Three-Phase PI Section Line : powerlib/Elements/Three-Phase PI Section Line  LConnTagsString=a|b|c  RConnTagsString=A|B|C  Frequency=50  Resistances=[ 0.274 0.959]  Inductances=[ 0.073 0.079]  Capacitances=[12.74e-9 7.751e-9]  Length=0.0025
      settings: SourceProductName=Simscape Electrical
  A : PMIOPort  Side=Left
  B : PMIOPort  Port=2  Side=Left
  C : PMIOPort  Port=3  Side=Left
  N : PMIOPort  Port=4  Side=Left
  a : PMIOPort  Port=5  Side=Right
  b : PMIOPort  Port=6  Side=Right
  c : PMIOPort  Port=7  Side=Right
  n : PMIOPort  Port=8  Side=Right
  connections:
  Pi Section Line/LConn1 -- N/RConn1
  Pi Section Line/RConn1 -- n/RConn1
  C/RConn1 -- Three-Phase PI Section Line/LConn3
  B/RConn1 -- Three-Phase PI Section Line/LConn2
  A/RConn1 -- Three-Phase PI Section Line/LConn1
  Three-Phase PI Section Line/RConn3 -- c/RConn1
  Three-Phase PI Section Line/RConn2 -- b/RConn1
  Three-Phase PI Section Line/RConn1 -- a/RConn1

== system LV_grid/L13/L1 ==
  Pi Section Line : powerlib/Elements/Pi Section Line  LConnTagsString=__new0  RConnTagsString=__new0  Frequency=50  Resistance=0.274  Inductance=0.073  Capacitance=12.74e-9  Length=0.0025  PiSections=1  Measurements=None
      settings: AttributesFormatString=\n  SourceProductName=Simscape Electrical  SourceProductBaseCode=PS
  Three-Phase PI Section Line : powerlib/Elements/Three-Phase PI Section Line  LConnTagsString=a|b|c  RConnTagsString=A|B|C  Frequency=50  Resistances=[ 0.274 0.959]  Inductances=[ 0.073 0.079]  Capacitances=[12.74e-9 7.751e-9]  Length=0.0025
      settings: SourceProductName=Simscape Electrical
  A : PMIOPort  Side=Left
  B : PMIOPort  Port=2  Side=Left
  C : PMIOPort  Port=3  Side=Left
  N : PMIOPort  Port=4  Side=Left
  a : PMIOPort  Port=5  Side=Right
  b : PMIOPort  Port=6  Side=Right
  c : PMIOPort  Port=7  Side=Right
  n : PMIOPort  Port=8  Side=Right
  connections:
  Pi Section Line/LConn1 -- N/RConn1
  Pi Section Line/RConn1 -- n/RConn1
  C/RConn1 -- Three-Phase PI Section Line/LConn3
  B/RConn1 -- Three-Phase PI Section Line/LConn2
  A/RConn1 -- Three-Phase PI Section Line/LConn1
  Three-Phase PI Section Line/RConn3 -- c/RConn1
  Three-Phase PI Section Line/RConn2 -- b/RConn1
  Three-Phase PI Section Line/RConn1 -- a/RConn1

== system LV_grid/L13/L2 ==
  Pi Section Line : powerlib/Elements/Pi Section Line  LConnTagsString=__new0  RConnTagsString=__new0  Frequency=50  Resistance=0.274  Inductance=0.073  Capacitance=12.74e-9  Length=0.0025  PiSections=1  Measurements=None
      settings: AttributesFormatString=\n  SourceProductName=Simscape Electrical  SourceProductBaseCode=PS
  Three-Phase PI Section Line : powerlib/Elements/Three-Phase PI Section Line  LConnTagsString=a|b|c  RConnTagsString=A|B|C  Frequency=50  Resistances=[ 0.274 0.959]  Inductances=[ 0.073 0.079]  Capacitances=[12.74e-9 7.751e-9]  Length=0.0025
      settings: SourceProductName=Simscape Electrical
  A : PMIOPort  Side=Left
  B : PMIOPort  Port=2  Side=Left
  C : PMIOPort  Port=3  Side=Left
  N : PMIOPort  Port=4  Side=Left
  a : PMIOPort  Port=5  Side=Right
  b : PMIOPort  Port=6  Side=Right
  c : PMIOPort  Port=7  Side=Right
  n : PMIOPort  Port=8  Side=Right
  connections:
  Pi Section Line/LConn1 -- N/RConn1
  Pi Section Line/RConn1 -- n/RConn1
  C/RConn1 -- Three-Phase PI Section Line/LConn3
  B/RConn1 -- Three-Phase PI Section Line/LConn2
  A/RConn1 -- Three-Phase PI Section Line/LConn1
  Three-Phase PI Section Line/RConn3 -- c/RConn1
  Three-Phase PI Section Line/RConn2 -- b/RConn1
  Three-Phase PI Section Line/RConn1 -- a/RConn1

== system LV_grid/L14/L1 ==
  Pi Section Line : powerlib/Elements/Pi Section Line  LConnTagsString=__new0  RConnTagsString=__new0  Frequency=50  Resistance=0.274  Inductance=0.073  Capacitance=12.74e-9  Length=0.0025  PiSections=1  Measurements=None
      settings: AttributesFormatString=\n  SourceProductName=Simscape Electrical  SourceProductBaseCode=PS
  Three-Phase PI Section Line : powerlib/Elements/Three-Phase PI Section Line  LConnTagsString=a|b|c  RConnTagsString=A|B|C  Frequency=50  Resistances=[ 0.274 0.959]  Inductances=[ 0.073 0.079]  Capacitances=[12.74e-9 7.751e-9]  Length=0.0025
      settings: SourceProductName=Simscape Electrical
  A : PMIOPort  Side=Left
  B : PMIOPort  Port=2  Side=Left
  C : PMIOPort  Port=3  Side=Left
  N : PMIOPort  Port=4  Side=Left
  a : PMIOPort  Port=5  Side=Right
  b : PMIOPort  Port=6  Side=Right
  c : PMIOPort  Port=7  Side=Right
  n : PMIOPort  Port=8  Side=Right
  connections:
  Pi Section Line/LConn1 -- N/RConn1
  Pi Section Line/RConn1 -- n/RConn1
  C/RConn1 -- Three-Phase PI Section Line/LConn3
  B/RConn1 -- Three-Phase PI Section Line/LConn2
  A/RConn1 -- Three-Phase PI Section Line/LConn1
  Three-Phase PI Section Line/RConn3 -- c/RConn1
  Three-Phase PI Section Line/RConn2 -- b/RConn1
  Three-Phase PI Section Line/RConn1 -- a/RConn1

== system LV_grid/L15/L1 ==
  Pi Section Line : powerlib/Elements/Pi Section Line  LConnTagsString=__new0  RConnTagsString=__new0  Frequency=50  Resistance=0.274  Inductance=0.073  Capacitance=12.74e-9  Length=0.0025  PiSections=1  Measurements=None
      settings: AttributesFormatString=\n  SourceProductName=Simscape Electrical  SourceProductBaseCode=PS
  Three-Phase PI Section Line : powerlib/Elements/Three-Phase PI Section Line  LConnTagsString=a|b|c  RConnTagsString=A|B|C  Frequency=50  Resistances=[ 0.274 0.959]  Inductances=[ 0.073 0.079]  Capacitances=[12.74e-9 7.751e-9]  Length=0.0025
      settings: SourceProductName=Simscape Electrical
  A : PMIOPort  Side=Left
  B : PMIOPort  Port=2  Side=Left
  C : PMIOPort  Port=3  Side=Left
  N : PMIOPort  Port=4  Side=Left
  a : PMIOPort  Port=5  Side=Right
  b : PMIOPort  Port=6  Side=Right
  c : PMIOPort  Port=7  Side=Right
  n : PMIOPort  Port=8  Side=Right
  connections:
  Pi Section Line/LConn1 -- N/RConn1
  Pi Section Line/RConn1 -- n/RConn1
  C/RConn1 -- Three-Phase PI Section Line/LConn3
  B/RConn1 -- Three-Phase PI Section Line/LConn2
  A/RConn1 -- Three-Phase PI Section Line/LConn1
  Three-Phase PI Section Line/RConn3 -- c/RConn1
  Three-Phase PI Section Line/RConn2 -- b/RConn1
  Three-Phase PI Section Line/RConn1 -- a/RConn1

== system LV_grid/L15/L2 ==
  Pi Section Line : powerlib/Elements/Pi Section Line  LConnTagsString=__new0  RConnTagsString=__new0  Frequency=50  Resistance=0.274  Inductance=0.073  Capacitance=12.74e-9  Length=0.0025  PiSections=1  Measurements=None
      settings: AttributesFormatString=\n  SourceProductName=Simscape Electrical  SourceProductBaseCode=PS
  Three-Phase PI Section Line : powerlib/Elements/Three-Phase PI Section Line  LConnTagsString=a|b|c  RConnTagsString=A|B|C  Frequency=50  Resistances=[ 0.274 0.959]  Inductances=[ 0.073 0.079]  Capacitances=[12.74e-9 7.751e-9]  Length=0.0025
      settings: SourceProductName=Simscape Electrical
  A : PMIOPort  Side=Left
  B : PMIOPort  Port=2  Side=Left
  C : PMIOPort  Port=3  Side=Left
  N : PMIOPort  Port=4  Side=Left
  a : PMIOPort  Port=5  Side=Right
  b : PMIOPort  Port=6  Side=Right
  c : PMIOPort  Port=7  Side=Right
  n : PMIOPort  Port=8  Side=Right
  connections:
  Pi Section Line/LConn1 -- N/RConn1
  Pi Section Line/RConn1 -- n/RConn1
  C/RConn1 -- Three-Phase PI Section Line/LConn3
  B/RConn1 -- Three-Phase PI Section Line/LConn2
  A/RConn1 -- Three-Phase PI Section Line/LConn1
  Three-Phase PI Section Line/RConn3 -- c/RConn1
  Three-Phase PI Section Line/RConn2 -- b/RConn1
  Three-Phase PI Section Line/RConn1 -- a/RConn1

== system LV_grid/L16/L1 ==
  Pi Section Line : powerlib/Elements/Pi Section Line  LConnTagsString=__new0  RConnTagsString=__new0  Frequency=50  Resistance=0.274  Inductance=0.073  Capacitance=12.74e-9  Length=0.0025  PiSections=1  Measurements=None
      settings: AttributesFormatString=\n  SourceProductName=Simscape Electrical  SourceProductBaseCode=PS
  Three-Phase PI Section Line : powerlib/Elements/Three-Phase PI Section Line  LConnTagsString=a|b|c  RConnTagsString=A|B|C  Frequency=50  Resistances=[ 0.274 0.959]  Inductances=[ 0.073 0.079]  Capacitances=[12.74e-9 7.751e-9]  Length=0.0025
      settings: SourceProductName=Simscape Electrical
  A : PMIOPort  Side=Left
  B : PMIOPort  Port=2  Side=Left
  C : PMIOPort  Port=3  Side=Left
  N : PMIOPort  Port=4  Side=Left
  a : PMIOPort  Port=5  Side=Right
  b : PMIOPort  Port=6  Side=Right
  c : PMIOPort  Port=7  Side=Right
  n : PMIOPort  Port=8  Side=Right
  connections:
  Pi Section Line/LConn1 -- N/RConn1
  Pi Section Line/RConn1 -- n/RConn1
  C/RConn1 -- Three-Phase PI Section Line/LConn3
  B/RConn1 -- Three-Phase PI Section Line/LConn2
  A/RConn1 -- Three-Phase PI Section Line/LConn1
  Three-Phase PI Section Line/RConn3 -- c/RConn1
  Three-Phase PI Section Line/RConn2 -- b/RConn1
  Three-Phase PI Section Line/RConn1 -- a/RConn1

== system LV_grid/L17/L1 ==
  Pi Section Line : powerlib/Elements/Pi Section Line  LConnTagsString=__new0  RConnTagsString=__new0  Frequency=50  Resistance=0.274  Inductance=0.073  Capacitance=12.74e-9  Length=0.0025  PiSections=1  Measurements=None
      settings: AttributesFormatString=\n  SourceProductName=Simscape Electrical  SourceProductBaseCode=PS
  Three-Phase PI Section Line : powerlib/Elements/Three-Phase PI Section Line  LConnTagsString=a|b|c  RConnTagsString=A|B|C  Frequency=50  Resistances=[ 0.274 0.959]  Inductances=[ 0.073 0.079]  Capacitances=[12.74e-9 7.751e-9]  Length=0.0025
      settings: SourceProductName=Simscape Electrical
  A : PMIOPort  Side=Left
  B : PMIOPort  Port=2  Side=Left
  C : PMIOPort  Port=3  Side=Left
  N : PMIOPort  Port=4  Side=Left
  a : PMIOPort  Port=5  Side=Right
  b : PMIOPort  Port=6  Side=Right
  c : PMIOPort  Port=7  Side=Right
  n : PMIOPort  Port=8  Side=Right
  connections:
  Pi Section Line/LConn1 -- N/RConn1
  Pi Section Line/RConn1 -- n/RConn1
  C/RConn1 -- Three-Phase PI Section Line/LConn3
  B/RConn1 -- Three-Phase PI Section Line/LConn2
  A/RConn1 -- Three-Phase PI Section Line/LConn1
  Three-Phase PI Section Line/RConn3 -- c/RConn1
  Three-Phase PI Section Line/RConn2 -- b/RConn1
  Three-Phase PI Section Line/RConn1 -- a/RConn1

== system LV_grid/L17/L2 ==
  Pi Section Line : powerlib/Elements/Pi Section Line  LConnTagsString=__new0  RConnTagsString=__new0  Frequency=50  Resistance=0.274  Inductance=0.073  Capacitance=12.74e-9  Length=0.0025  PiSections=1  Measurements=None
      settings: AttributesFormatString=\n  SourceProductName=Simscape Electrical  SourceProductBaseCode=PS
  Three-Phase PI Section Line : powerlib/Elements/Three-Phase PI Section Line  LConnTagsString=a|b|c  RConnTagsString=A|B|C  Frequency=50  Resistances=[ 0.274 0.959]  Inductances=[ 0.073 0.079]  Capacitances=[12.74e-9 7.751e-9]  Length=0.0025
      settings: SourceProductName=Simscape Electrical
  A : PMIOPort  Side=Left
  B : PMIOPort  Port=2  Side=Left
  C : PMIOPort  Port=3  Side=Left
  N : PMIOPort  Port=4  Side=Left
  a : PMIOPort  Port=5  Side=Right
  b : PMIOPort  Port=6  Side=Right
  c : PMIOPort  Port=7  Side=Right
  n : PMIOPort  Port=8  Side=Right
  connections:
  Pi Section Line/LConn1 -- N/RConn1
  Pi Section Line/RConn1 -- n/RConn1
  C/RConn1 -- Three-Phase PI Section Line/LConn3
  B/RConn1 -- Three-Phase PI Section Line/LConn2
  A/RConn1 -- Three-Phase PI Section Line/LConn1
  Three-Phase PI Section Line/RConn3 -- c/RConn1
  Three-Phase PI Section Line/RConn2 -- b/RConn1
  Three-Phase PI Section Line/RConn1 -- a/RConn1

== system LV_grid/L17/L3 ==
  Pi Section Line : powerlib/Elements/Pi Section Line  LConnTagsString=__new0  RConnTagsString=__new0  Frequency=50  Resistance=0.274  Inductance=0.073  Capacitance=12.74e-9  Length=0.0025  PiSections=1  Measurements=None
      settings: AttributesFormatString=\n  SourceProductName=Simscape Electrical  SourceProductBaseCode=PS
  Three-Phase PI Section Line : powerlib/Elements/Three-Phase PI Section Line  LConnTagsString=a|b|c  RConnTagsString=A|B|C  Frequency=50  Resistances=[ 0.274 0.959]  Inductances=[ 0.073 0.079]  Capacitances=[12.74e-9 7.751e-9]  Length=0.0025
      settings: SourceProductName=Simscape Electrical
  A : PMIOPort  Side=Left
  B : PMIOPort  Port=2  Side=Left
  C : PMIOPort  Port=3  Side=Left
  N : PMIOPort  Port=4  Side=Left
  a : PMIOPort  Port=5  Side=Right
  b : PMIOPort  Port=6  Side=Right
  c : PMIOPort  Port=7  Side=Right
  n : PMIOPort  Port=8  Side=Right
  connections:
  Pi Section Line/LConn1 -- N/RConn1
  Pi Section Line/RConn1 -- n/RConn1
  C/RConn1 -- Three-Phase PI Section Line/LConn3
  B/RConn1 -- Three-Phase PI Section Line/LConn2
  A/RConn1 -- Three-Phase PI Section Line/LConn1
  Three-Phase PI Section Line/RConn3 -- c/RConn1
  Three-Phase PI Section Line/RConn2 -- b/RConn1
  Three-Phase PI Section Line/RConn1 -- a/RConn1

== system LV_grid/L18/L1 ==
  Pi Section Line : powerlib/Elements/Pi Section Line  LConnTagsString=__new0  RConnTagsString=__new0  Frequency=50  Resistance=0.274  Inductance=0.073  Capacitance=12.74e-9  Length=0.0025  PiSections=1  Measurements=None
      settings: AttributesFormatString=\n  SourceProductName=Simscape Electrical  SourceProductBaseCode=PS
  Three-Phase PI Section Line : powerlib/Elements/Three-Phase PI Section Line  LConnTagsString=a|b|c  RConnTagsString=A|B|C  Frequency=50  Resistances=[ 0.274 0.959]  Inductances=[ 0.073 0.079]  Capacitances=[12.74e-9 7.751e-9]  Length=0.0025
      settings: SourceProductName=Simscape Electrical
  A : PMIOPort  Side=Left
  B : PMIOPort  Port=2  Side=Left
  C : PMIOPort  Port=3  Side=Left
  N : PMIOPort  Port=4  Side=Left
  a : PMIOPort  Port=5  Side=Right
  b : PMIOPort  Port=6  Side=Right
  c : PMIOPort  Port=7  Side=Right
  n : PMIOPort  Port=8  Side=Right
  connections:
  Pi Section Line/LConn1 -- N/RConn1
  Pi Section Line/RConn1 -- n/RConn1
  C/RConn1 -- Three-Phase PI Section Line/LConn3
  B/RConn1 -- Three-Phase PI Section Line/LConn2
  A/RConn1 -- Three-Phase PI Section Line/LConn1
  Three-Phase PI Section Line/RConn3 -- c/RConn1
  Three-Phase PI Section Line/RConn2 -- b/RConn1
  Three-Phase PI Section Line/RConn1 -- a/RConn1

== system LV_grid/L18/L2 ==
  Pi Section Line : powerlib/Elements/Pi Section Line  LConnTagsString=__new0  RConnTagsString=__new0  Frequency=50  Resistance=0.274  Inductance=0.073  Capacitance=12.74e-9  Length=0.0025  PiSections=1  Measurements=None
      settings: AttributesFormatString=\n  SourceProductName=Simscape Electrical  SourceProductBaseCode=PS
  Three-Phase PI Section Line : powerlib/Elements/Three-Phase PI Section Line  LConnTagsString=a|b|c  RConnTagsString=A|B|C  Frequency=50  Resistances=[ 0.274 0.959]  Inductances=[ 0.073 0.079]  Capacitances=[12.74e-9 7.751e-9]  Length=0.0025
      settings: SourceProductName=Simscape Electrical
  A : PMIOPort  Side=Left
  B : PMIOPort  Port=2  Side=Left
  C : PMIOPort  Port=3  Side=Left
  N : PMIOPort  Port=4  Side=Left
  a : PMIOPort  Port=5  Side=Right
  b : PMIOPort  Port=6  Side=Right
  c : PMIOPort  Port=7  Side=Right
  n : PMIOPort  Port=8  Side=Right
  connections:
  Pi Section Line/LConn1 -- N/RConn1
  Pi Section Line/RConn1 -- n/RConn1
  C/RConn1 -- Three-Phase PI Section Line/LConn3
  B/RConn1 -- Three-Phase PI Section Line/LConn2
  A/RConn1 -- Three-Phase PI Section Line/LConn1
  Three-Phase PI Section Line/RConn3 -- c/RConn1
  Three-Phase PI Section Line/RConn2 -- b/RConn1
  Three-Phase PI Section Line/RConn1 -- a/RConn1

== system LV_grid/L19/L1 ==
  Pi Section Line : powerlib/Elements/Pi Section Line  LConnTagsString=__new0  RConnTagsString=__new0  Frequency=50  Resistance=0.274  Inductance=0.073  Capacitance=12.74e-9  Length=0.0025  PiSections=1  Measurements=None
      settings: AttributesFormatString=\n  SourceProductName=Simscape Electrical  SourceProductBaseCode=PS
  Three-Phase PI Section Line : powerlib/Elements/Three-Phase PI Section Line  LConnTagsString=a|b|c  RConnTagsString=A|B|C  Frequency=50  Resistances=[ 0.274 0.959]  Inductances=[ 0.073 0.079]  Capacitances=[12.74e-9 7.751e-9]  Length=0.0025
      settings: SourceProductName=Simscape Electrical
  A : PMIOPort  Side=Left
  B : PMIOPort  Port=2  Side=Left
  C : PMIOPort  Port=3  Side=Left
  N : PMIOPort  Port=4  Side=Left
  a : PMIOPort  Port=5  Side=Right
  b : PMIOPort  Port=6  Side=Right
  c : PMIOPort  Port=7  Side=Right
  n : PMIOPort  Port=8  Side=Right
  connections:
  Pi Section Line/LConn1 -- N/RConn1
  Pi Section Line/RConn1 -- n/RConn1
  C/RConn1 -- Three-Phase PI Section Line/LConn3
  B/RConn1 -- Three-Phase PI Section Line/LConn2
  A/RConn1 -- Three-Phase PI Section Line/LConn1
  Three-Phase PI Section Line/RConn3 -- c/RConn1
  Three-Phase PI Section Line/RConn2 -- b/RConn1
  Three-Phase PI Section Line/RConn1 -- a/RConn1
